simulink model "delay"  (R2016a)
settings: Solver=FixedStepDiscrete  StartTime=0.0  StopTime=10.0  RelTol=1e-3
libraries: rvs x7
settings Model: Creator=Arthur  LastModifiedBy=arthur
settings DataIOCC: LimitDataPoints=on  SaveFormat=Array
settings DebuggingCC: SolverPrmCheckMsg=warning
settings HardwareCC: ProdBitPerPointer=32  ProdLargestAtomicFloat=None  ProdIntDivRoundTo=Undefined  ProdEndianess=Unspecified  ProdWordSize=32  ProdHWDeviceType=32-bit Generic
settings ModelReferenceCC: PropagateSignalLabelsOutOfModel=off
settings ConfigComp: CovModelRefEnable=Off  CovSFcnEnable=off

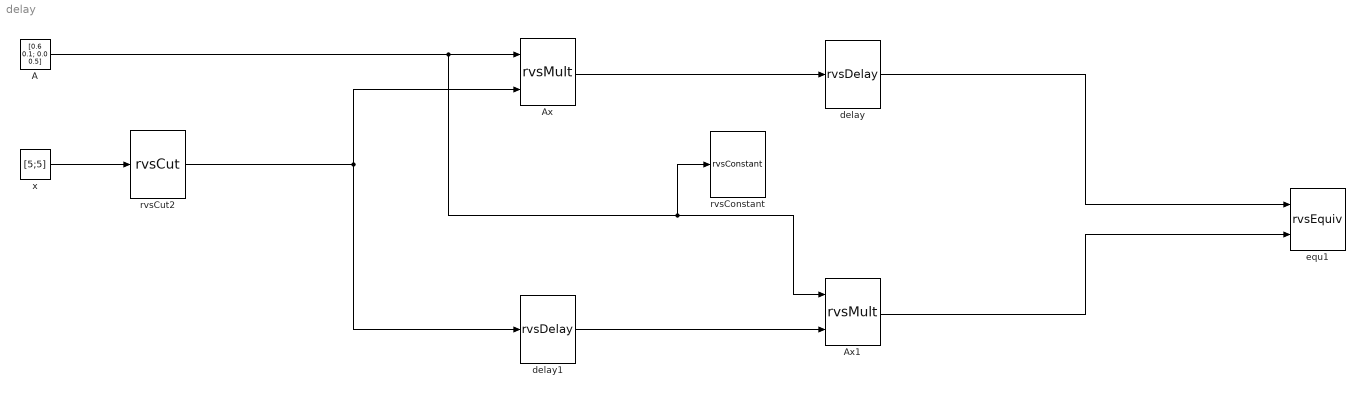
== system delay ==
  A : Constant  Value=[0.6 0.1; 0.0 0.5]
  Ax : rvs/rvsMult
  Ax1 : rvs/rvsMult
  delay : rvs/rvsDelay  xInit=[0;0]
  delay1 : rvs/rvsDelay  xInit=[1;0]
  equ1 : rvs/rvsEquiv  tol=1e-9  nIgnoreSteps=1
  rvsConstant : rvs/rvsConstant
  rvsCut2 : rvs/rvsCut
  x : Constant  Value=[5;5]
  wires:
  Ax/1 -> delay/1
  A/1 -> rvsConstant/1, Ax1/1, Ax/1
  x/1 -> rvsCut2/1
  rvsCut2/1 -> delay1/1, Ax/2
  delay1/1 -> Ax1/2
  delay/1 -> equ1/1
  Ax1/1 -> equ1/2
